simulink model "Model_LAB3_ssSYSTEM_robust"  (R2024b)
settings: Solver=ode45  StartTime=0.0  StopTime=5  RelTol=1e-2
values from neighbouring files (symbols this model uses):
  H1_den = [1, 2*delta1*omega_c, omega_c^2]    [Controller_LAB3_ssVAR.m]
  H1_num = [omega_c^2 0]    [Controller_LAB3_ssVAR.m]
undefined symbols (not defined in the file or in its folder): degs2rpm, pulse2deg, sens
settings Model: Creator=Federico Bergami  LastModifiedBy=Buton

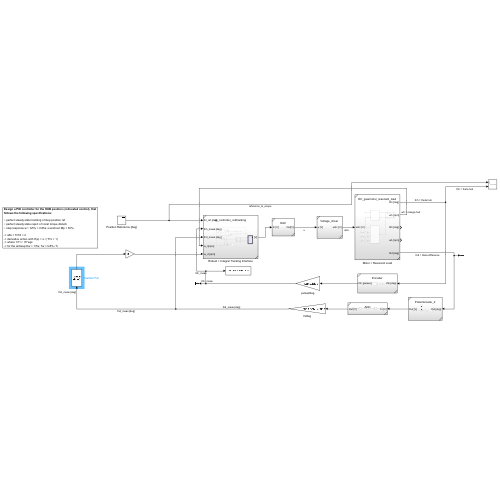
[thumbnail: Simulink's stored preview of the top-level diagram]
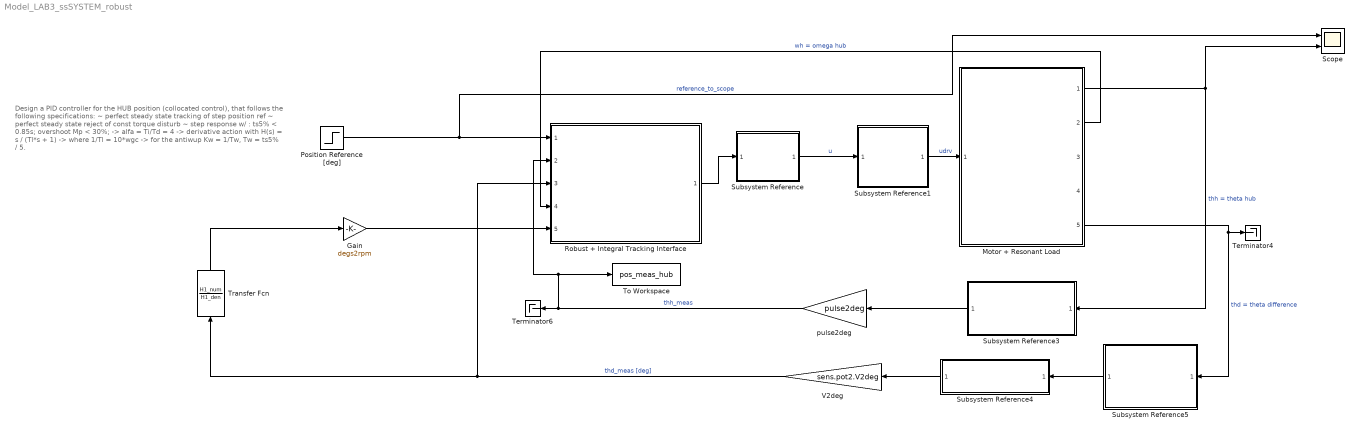
== system Model_LAB3_ssSYSTEM_robust ==
  note: Design a PID controller for the HUB position (collocated control), that
      | follows the following specifications:
      |
      | ~ perfect steady state tracking of step position ref
      | ~ perfect steady state reject of const torque disturb
      | ~ step response w/ : ts5% < 0.85s; overshoot Mp < 30%;
      |
      | -> alfa = Ti/Td = 4
      | -> derivative action with H(s) = s / (Tl*s + 1)
      | -> where 1/Tl = 10*wgc
      | -> for the antiwup Kw = 1/Tw, Tw = ts5% / 5.
  Gain : Gain  Gain=degs2rpm
  Motor + Resonant Load : Subsystem  ReferencedSubsystem=DC_gearmotor_resonant_load
  Position Reference [deg] : Step  After=50  SampleTime=0
  Robust + Integral Tracking Interface : Subsystem  ReferencedSubsystem=ss_controller_robtracking
  Scope : Scope  NumInputPorts=2
  Subsystem Reference : Subsystem  ReferencedSubsystem=DAC
  Subsystem Reference1 : Subsystem  ReferencedSubsystem=Voltage_driver
  Subsystem Reference3 : Subsystem  ReferencedSubsystem=Encoder
  Subsystem Reference4 : Subsystem  ReferencedSubsystem=ADC
  Subsystem Reference5 : Subsystem  ReferencedSubsystem=Potentiometer_2
  Terminator4 : Terminator
  Terminator6 : Terminator
  To Workspace : ToWorkspace  VariableName=pos_meas_hub  SaveFormat=Timeseries  SampleTime=-1
  Transfer Fcn : TransferFcn  Numerator=H1_num  Denominator=H1_den
  V2deg : Gain  Gain=sens.pot2.V2deg
  pulse2deg : Gain  Gain=pulse2deg
  wires:
  Subsystem Reference/1 -> Subsystem Reference1/1  "u"
  Subsystem Reference3/1 -> pulse2deg/1
  Motor + Resonant Load/5 -> Subsystem Reference5/1, Terminator4/1  "thd = theta difference"
  Motor + Resonant Load/1 -> Scope/2, Subsystem Reference3/1  "thh = theta hub"
  Position Reference [deg]/1 -> Robust + Integral Tracking Interface/1, Scope/1  "reference_to_scope"
  pulse2deg/1 -> Terminator6/1, Robust + Integral Tracking Interface/2, To Workspace/1  "thh_meas"
  Transfer Fcn/1 -> Gain/1
  V2deg/1 -> Robust + Integral Tracking Interface/3, Transfer Fcn/1  "thd_meas [deg]"
  Motor + Resonant Load/2 -> Robust + Integral Tracking Interface/4  "wh = omega hub"
  Subsystem Reference4/1 -> V2deg/1
  Subsystem Reference5/1 -> Subsystem Reference4/1
  Subsystem Reference1/1 -> Motor + Resonant Load/1  "udrv"
  Gain/1 -> Robust + Integral Tracking Interface/5
  Robust + Integral Tracking Interface/1 -> Subsystem Reference/1
